simulink model "Controlador_Mamdani"  (R2020b)
settings: Solver=ode3  StartTime=0.0  StopTime=200  FixedStep=0.1  RelTol=1e-3
undefined symbols (not defined in the file or in its folder): Angular, Linear
libraries: robotlib x11, fuzblock x1, robotcorelib x1
settings Model: EnablePacing=on  Creator=pizarro  LastModifiedBy=celuc
settings DataIOCC: ReturnWorkspaceOutputs=off
settings SFSimCC: CustomCodeUndefinedFunction=UseInterfaceOnly

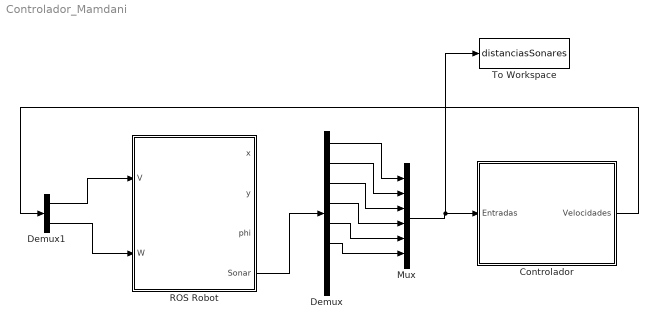
== system Controlador_Mamdani ==
  Controlador : Subsystem
  Demux : Demux  Outputs=8
  Demux1 : Demux  Outputs=2
  Mux : Mux  Inputs=6
  ROS Robot : Subsystem
  To Workspace : ToWorkspace  VariableName=distanciasSonares  SaveFormat=Structure With Time  SampleTime=-1
  wires:
  ROS Robot/4(Sonar) -> Demux/1
  Mux/1 -> To Workspace/1, Controlador/1(Entradas)
  Demux/1 -> Mux/1
  Demux/3 -> Mux/3
  Demux/4 -> Mux/4
  Demux/6 -> Mux/6
  Demux1/1 -> ROS Robot/1(V)
  Demux1/2 -> ROS Robot/2(W)
  Controlador/1(Velocidades) -> Demux1/1
  Demux/5 -> Mux/5
  Demux/2 -> Mux/2

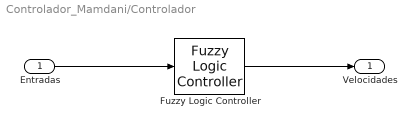
== system Controlador_Mamdani/Controlador ==
  Entradas : Inport
  Fuzzy Logic Controller : fuzblock/Fuzzy Logic  Controller  FIS='ControladorMamdani.fis'  OutputSampleNumber=101  DataType=double  FuzzifiedInputs=off  RuleFiringStrengths=off  RuleOutputs=off  AggregatedOutputs=off  SimulateUsing=Interpreted execution  OutOfRangeInputValueMessage=warning  NoRuleFiredMessage=warning  EmptyOutputFuzzySetMessage=warning
  Velocidades : Outport  VectorParamsAs1DForOutWhenUnconnected=off
  wires:
  Fuzzy Logic Controller/1 -> Velocidades/1
  Entradas/1 -> Fuzzy Logic Controller/1

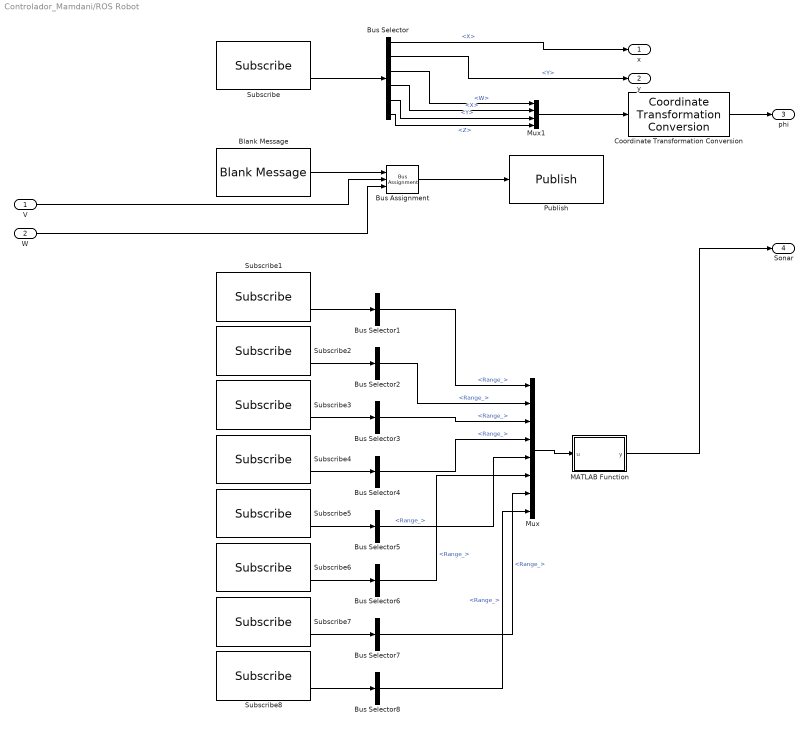
== system Controlador_Mamdani/ROS Robot ==
  V : Inport
  W : Inport  Port=2
  Blank Message : robotlib/Blank Message  messageClass=Message  entityType=geometry_msgs/Twist  messageType=geometry_msgs/Twist  SampleTime=-1  legacyBusStruct=off
  Bus Assignment : BusAssignment  AssignedSignals=Linear.X,Angular.Z
  Bus Selector : BusSelector  OutputSignals=Pose.Pose.Position.X,Pose.Pose.Position.Y,Pose.Pose.Orientation.W,Pose.Pose.Orientation.X,Pose.Pose.Orientation.Y,Pose.Pose.Orientation.Z
  Bus Selector{1..8} (8 alike) : BusSelector  OutputSignals=Range_
  Coordinate Transformation Conversion : robotcorelib/Coordinate Transformation Conversion  InputRepresentation=Quaternion  InputEulerSequence=ZYX  ShowTrVecInputPort=on  OutputRepresentation=Euler Angles  OutputEulerSequence=ZYX  ShowTrVecOutputPort=on  SimulateUsing=Interpreted execution
      settings: SourceProductBaseCode=NV,RO,RR,UV
  MATLAB Function : MATLAB Function  TreatAsAtomicUnit=on
  Mux : Mux  Inputs=8
  Mux1 : Mux
  Publish : robotlib/Publish  topicSource=Select from ROS network  topic=/robot0/cmd_vel  messageType=geometry_msgs/Twist  legacyBusStruct=off  messageQueueLength=1
  Subscribe : robotlib/Subscribe  topicSource=Select from ROS network  topic=/robot0/odom  messageType=nav_msgs/Odometry  SampleTime=-1  legacyBusStruct=off  messageQueueLength=1
  Subscribe1 : robotlib/Subscribe  topicSource=Select from ROS network  topic=/robot0/sonar_0  messageType=sensor_msgs/Range  SampleTime=-1  legacyBusStruct=off  messageQueueLength=1
  Subscribe2 : robotlib/Subscribe  topicSource=Select from ROS network  topic=/robot0/sonar_1  messageType=sensor_msgs/Range  SampleTime=-1  legacyBusStruct=off  messageQueueLength=1
  Subscribe3 : robotlib/Subscribe  topicSource=Select from ROS network  topic=/robot0/sonar_2  messageType=sensor_msgs/Range  SampleTime=-1  legacyBusStruct=off  messageQueueLength=1
  Subscribe4 : robotlib/Subscribe  topicSource=Select from ROS network  topic=/robot0/sonar_3  messageType=sensor_msgs/Range  SampleTime=-1  legacyBusStruct=off  messageQueueLength=1
  Subscribe5 : robotlib/Subscribe  topicSource=Select from ROS network  topic=/robot0/sonar_4  messageType=sensor_msgs/Range  SampleTime=-1  legacyBusStruct=off  messageQueueLength=1
  Subscribe6 : robotlib/Subscribe  topicSource=Select from ROS network  topic=/robot0/sonar_5  messageType=sensor_msgs/Range  SampleTime=-1  legacyBusStruct=off  messageQueueLength=1
  Subscribe7 : robotlib/Subscribe  topicSource=Select from ROS network  topic=/robot0/sonar_6  messageType=sensor_msgs/Range  SampleTime=-1  legacyBusStruct=off  messageQueueLength=1
  Subscribe8 : robotlib/Subscribe  topicSource=Select from ROS network  topic=/robot0/sonar_7  messageType=sensor_msgs/Range  SampleTime=-1  legacyBusStruct=off  messageQueueLength=1
  x : Outport  VectorParamsAs1DForOutWhenUnconnected=off
  y : Outport  Port=2  VectorParamsAs1DForOutWhenUnconnected=off
  phi : Outport  Port=3  VectorParamsAs1DForOutWhenUnconnected=off
  Sonar : Outport  Port=4  VectorParamsAs1DForOutWhenUnconnected=off
  wires:
  Bus Selector/1 -> x/1  "<X>"
  Blank Message/1 -> Bus Assignment/1
  Subscribe/2 -> Bus Selector/1
  Bus Assignment/1 -> Publish/1
  Bus Selector/2 -> y/1  "<Y>"
  Subscribe1/2 -> Bus Selector1/1
  V/1 -> Bus Assignment/2
  W/1 -> Bus Assignment/3
  Subscribe2/2 -> Bus Selector2/1
  Subscribe3/2 -> Bus Selector3/1
  Subscribe5/2 -> Bus Selector5/1
  Subscribe4/2 -> Bus Selector4/1
  Subscribe6/2 -> Bus Selector6/1
  Subscribe7/2 -> Bus Selector7/1
  Bus Selector1/1 -> Mux/1  "<Range_>"
  Bus Selector2/1 -> Mux/2  "<Range_>"
  Bus Selector3/1 -> Mux/3  "<Range_>"
  Bus Selector4/1 -> Mux/4  "<Range_>"
  Bus Selector5/1 -> Mux/5  "<Range_>"
  Bus Selector6/1 -> Mux/6  "<Range_>"
  Bus Selector7/1 -> Mux/7  "<Range_>"
  Subscribe8/2 -> Bus Selector8/1
  Bus Selector8/1 -> Mux/8  "<Range_>"
  Bus Selector/3 -> Mux1/1  "<W>"
  Bus Selector/4 -> Mux1/2  "<X>"
  Bus Selector/5 -> Mux1/3  "<Y>"
  Bus Selector/6 -> Mux1/4  "<Z>"
  Mux1/1 -> Coordinate Transformation Conversion/1
  Coordinate Transformation Conversion/1 -> phi/1
  Mux/1 -> MATLAB Function/1(u)
  MATLAB Function/1(y) -> Sonar/1

== matlab function Controlador_Mamdani/ROS Robot/MATLAB Function ==
  data: u input; y output
function y = fcn(u)
u(isinf(u))=5.0;
y = u;
